simulink model "sim_6a_dis"  (R2022b)
settings: Solver=ode4  StartTime=0.0  StopTime=8.0  FixedStep=tstep  RelTol=1e-3
undefined symbols (not defined in the file): den, num
settings Model: Creator=dipte  LastModifiedBy=dipte
settings DataIOCC: ReturnWorkspaceOutputs=off

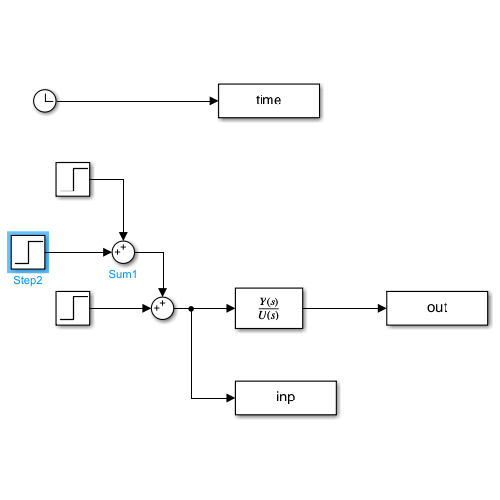
[thumbnail: Simulink's stored preview of the top-level diagram]
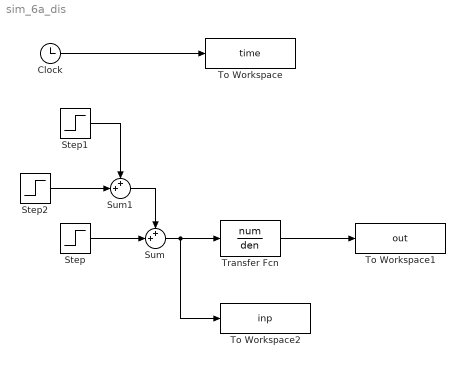
== system sim_6a_dis ==
  Clock : Clock
  Step : Step  Time=0  SampleTime=0
  Step1 : Step  Time=0  SampleTime=0
  Step2 : Step  Time=4  SampleTime=0
  Sum : Sum  Inputs=++|
  Sum1 : Sum  Inputs=++|
  To Workspace : ToWorkspace  VariableName=time  SampleTime=-1
      settings: Save2DSignal=2-D array (concatenate along first dimension)
  To Workspace1 : ToWorkspace  VariableName=out  SampleTime=-1
      settings: Save2DSignal=2-D array (concatenate along first dimension)
  To Workspace2 : ToWorkspace  VariableName=inp  SampleTime=-1
      settings: Save2DSignal=2-D array (concatenate along first dimension)
  Transfer Fcn : TransferFcn  Numerator=num  Denominator=den
  wires:
  Clock/1 -> To Workspace/1
  Transfer Fcn/1 -> To Workspace1/1
  Sum/1 -> To Workspace2/1, Transfer Fcn/1
  Step/1 -> Sum/2
  Sum1/1 -> Sum/1
  Step2/1 -> Sum1/2
  Step1/1 -> Sum1/1
